simulink model "harness"  (R2021b)
settings: Solver=VariableStepAuto  StartTime=0.0  StopTime=inf  FixedStep=1/10  RelTol=1e-3
libraries: simulink x1
settings Model: PacingRate=3  Creator=DAUIN-Win10  LastModifiedBy=alexf

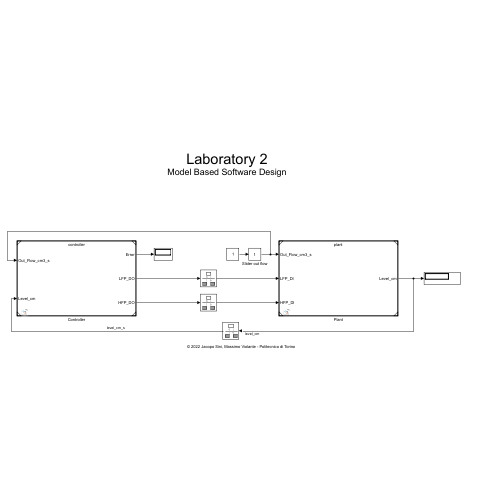
[thumbnail: Simulink's stored preview of the top-level diagram]
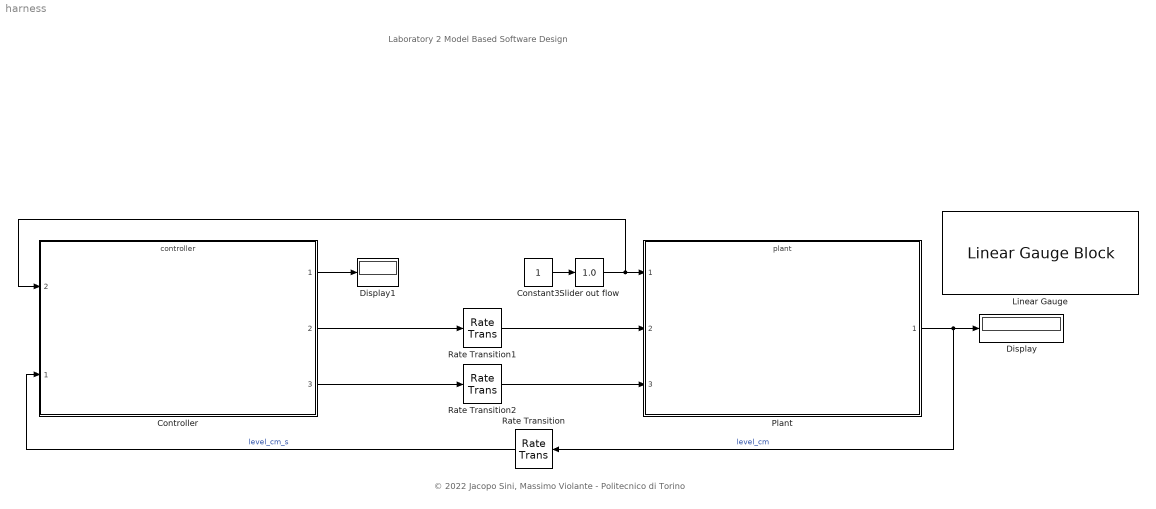
== system harness ==
  note: © 2022 Jacopo Sini, Massimo Violante - Politecnico di Torino
  note: Laboratory 2
      | Model Based Software Design
  Constant3 : Constant
  Controller : ModelReference  ModelNameDialog=controller  SimulationMode=Normal  ModelReferenceVersion=2.30
      settings: PortSchema="{\"entries\":[{\"content\":{\"sides\":[{\"content\":{\"connectorIds\":[\"In2\",\"In1\"]},\"type\":\"ConnectorPlacement.EquallySpacedRectSide\",\"uuid\":\"5e260b81-e1ce-497c-8572-ac5c2182ee27\"},{\"content\":{\"connectorIds\":[\"Out1\",\"Out2\",\"Out3\"],\"side\":\"RIGHT\"},\"type\":\"ConnectorPlacement.EquallySpacedRectSide\",\"uuid\":\"4325f63c-e453-4c79-ab01-1476da99aa25\"},{\"content\":{\"connectorIds\":[],\"side\":\"TOP\"},\"type\":\"ConnectorPlacement.EquallySpacedRectSide\",\"uuid\":\"dba88bac-0f95-4a98-ba3b-c40df5616f56\"}]},\"type\":\"ConnectorPlacement.EquallySpacedConnector\",\"uuid\":\"6943e10d-f3b0-4fd8-a142-b6b49e651f90\"}],\"packageUris\":[\"http://schema.mathworks.com/mf0/Connector/R2020b\"],\"version\":\"1.0\"}"
  Display : Display
  Display1 : Display
  Linear Gauge : LinearGaugeBlock  ScaleMax=220
  Plant : ModelReference  ModelNameDialog=plant  SimulationMode=Normal  ModelReferenceVersion=2.1
  Rate Transition : RateTransition
  Rate Transition1 : RateTransition
  Rate Transition2 : RateTransition
  Slider out flow : simulink/Math Operations/Slider Gain  gain=1.0  low=0  high=1
  wires:
  Plant/1 -> Rate Transition/1, Display/1  "level_cm"
  Slider out flow/1 -> Controller/2, Plant/1
  Constant3/1 -> Slider out flow/1
  Controller/1 -> Display1/1
  Rate Transition1/1 -> Plant/2
  Rate Transition2/1 -> Plant/3
  Rate Transition/1 -> Controller/1  "level_cm_s"
  Controller/3 -> Rate Transition2/1
  Controller/2 -> Rate Transition1/1
